simulink model "Simulink_Pendu_v1"  (R2019a)
settings: Solver=FixedStepAuto  StartTime=0.0  StopTime=inf  RelTol=1e-3  EnableMultiTasking=on
libraries: eeGeneralControl x3, cm_custom x2, simulink x1
settings Model: SimulationMode=external  Creator=Ng Wee Shen  LastModifiedBy=rng
settings SolverCC: PositivePriorityOrder=on  AutoInsertRateTranBlk=on
settings DataIOCC: ReturnWorkspaceOutputs=off
settings OptimizationCC: EnhancedBackFolding=on  PassReuseOutputArgsAs=Individual arguments  MaxStackSize=64  OptimizeBlockOrder=speed  DifferentSizesBufferReuse=on
settings DebuggingCC: TimeAdjustmentMsg=warning  SingleTaskRateTransMsg=warning  ParameterTunabilityLossMsg=error  SFcnCompatibilityMsg=warning  ArithmeticOperatorsInVariantConditions=warning
settings HardwareCC: ProdBitPerPointer=32  ProdBitPerSizeT=32  ProdBitPerPtrDiffT=32  ProdLargestAtomicInteger=Long  ProdLargestAtomicFloat=Double  ProdWordSize=32  ProdHWDeviceType=ARM Compatible->ARM Cortex
settings SFSimCC: MATLABDynamicMemAlloc=off
settings RTWCC: SystemTargetFile=ert.tlc  HardwareBoard=Raspberry Pi  TLCOptions="-aInlineSetEventsForThisBaseRateFcn=TLC_FALSE -aSuppressMultiTaskScheduler=TLC_FALSE  -aRateBasedStepFcn=0"  TemplateMakefile=ert_default_tmf  Toolchain=GNU GCC Raspberry Pi  BuildConfiguration=Specify  IncludeHyperlinkInReport=on  TargetLang=C++
settings CodeAppCC: ForceParamTrailComments=on  IgnoreCustomStorageClasses=off  OperatorAnnotations=on  SimulinkDataObjDesc=on  SFDataObjDesc=on  InsertBlockDesc=on
settings ERTTargetCC: TargetLangStandard=C++03 (ISO)  SupportContinuousTime=on  SupportVariableSizeSignals=on  ExtMode=on  ExtModeMexArgs='192.168.0.173' 1 17725

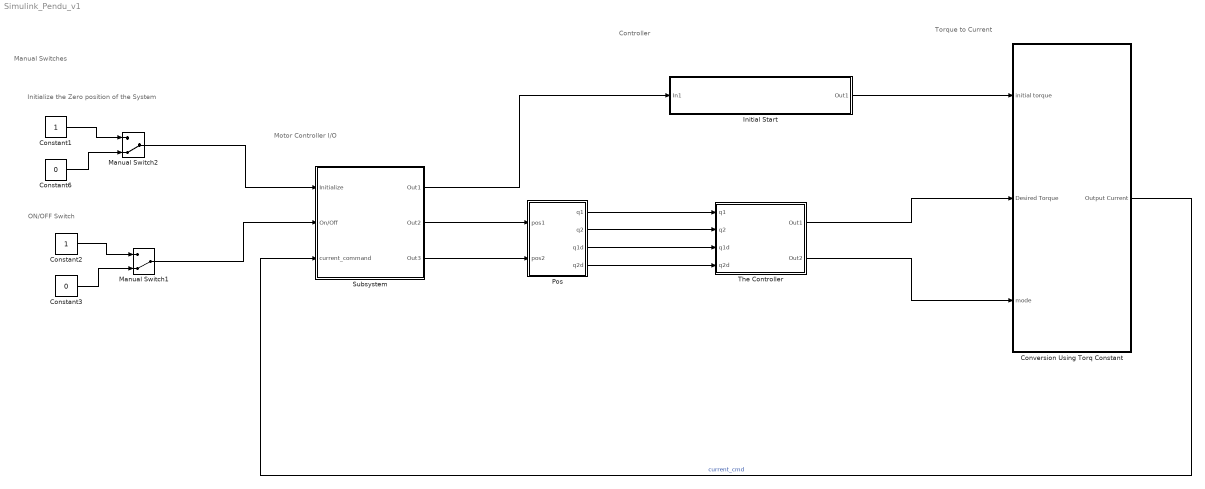
== system Simulink_Pendu_v1 ==
  note: Torque to Current
  note: Controller
  note: Motor Controller I/O
  note: Manual Switches
  note: ON/OFF Switch
  note: Initialize the Zero position of the System
  Constant1 : Constant
  Constant2 : Constant
  Constant3 : Constant  Value=0
  Constant6 : Constant  Value=0
  Conversion Using Torq Constant : Subsystem
  Initial Start : Subsystem
  Manual Switch1 : ManualSwitch  CurrentSetting=0
  Manual Switch2 : ManualSwitch  CurrentSetting=0
  Pos : Subsystem
  Subsystem : Subsystem
  The Controller : Subsystem
  wires:
  Constant1/1 -> Manual Switch2/1
  Constant6/1 -> Manual Switch2/2
  Initial Start/1(Out1) -> Conversion Using Torq Constant/1(initial torque)
  Pos/1(q1) -> The Controller/1(q1)
  Pos/2(q2) -> The Controller/2(q2)
  Pos/3(q1d) -> The Controller/3(q1d)
  Pos/4(q2d) -> The Controller/4(q2d)
  The Controller/1(Out1) -> Conversion Using Torq Constant/2(Desired Torque)
  The Controller/2(Out2) -> Conversion Using Torq Constant/3(" mode ")
  Manual Switch2/1 -> Subsystem/1(Initialize)
  Subsystem/1(Out1) -> Initial Start/1(In1)
  Subsystem/2(Out2) -> Pos/1(pos1)
  Subsystem/3(Out3) -> Pos/2(pos2)
  Constant2/1 -> Manual Switch1/1
  Constant3/1 -> Manual Switch1/2
  Manual Switch1/1 -> Subsystem/2(On/Off)
  Conversion Using Torq Constant/1(Output Current) -> Subsystem/3(current_command)  "current_cmd"

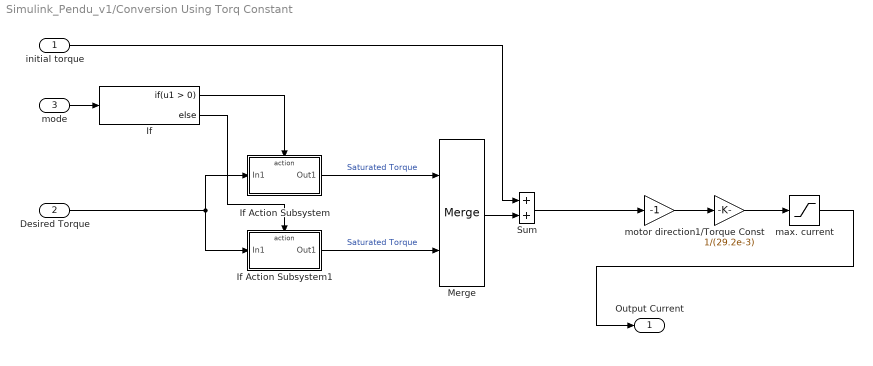
== system Simulink_Pendu_v1/Conversion Using Torq Constant ==
  initial torque : Inport
  Desired Torque : Inport  Port=2
  " mode " : Inport  Port=3
  1/Torque Const : Gain  Gain=1/(29.2e-3)  OutDataTypeStr=Inherit: Same as input
  If : If
  If Action Subsystem : Subsystem  TreatAsAtomicUnit=on
  If Action Subsystem1 : Subsystem  TreatAsAtomicUnit=on
  Merge : Merge
  Sum : Sum
  max. current : Saturate  UpperLimit=3  LowerLimit=-3  LinearizeAsGain=off
  motor direction : Gain  Gain=-1  OutDataTypeStr=Inherit: Same as input
  Output Current : Outport
  wires:
  motor direction/1 -> 1/Torque Const/1
  1/Torque Const/1 -> max. current/1
  " mode "/1 -> If/1
  Desired Torque/1 -> If Action Subsystem/1(In1), If Action Subsystem1/1(In1)
  If Action Subsystem/1(Out1) -> Merge/1  "Saturated Torque"
  If Action Subsystem1/1(Out1) -> Merge/2  "Saturated Torque"
  If/1 -> If Action Subsystem/Action
  If/2 -> If Action Subsystem1/Action
  Merge/1 -> Sum/2
  Sum/1 -> motor direction/1
  initial torque/1 -> Sum/1
  max. current/1 -> Output Current/1

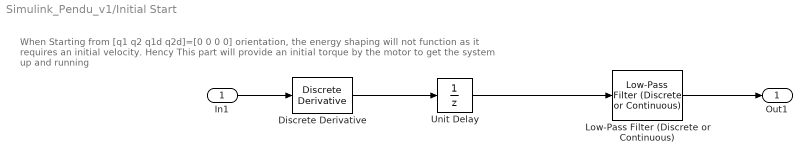
== system Simulink_Pendu_v1/Initial Start ==
  note: When Starting from [q1 q2 q1d q2d]=[0 0 0 0] orientation, the energy shaping will not function as it requires an initial velocity. Hency This part will provide an initial torque by the motor to get the system up and running
  In1 : Inport
  Discrete Derivative : simulink/Discrete/Discrete Derivative  gainval=1.0  ICPrevScaledInput=0.0  OutMin=[]  OutMax=[]  OutDataType=fixdt(1, 16)  OutScaling=2^-10  DoSatur=off
  Low-Pass Filter (Discrete or Continuous) : eeGeneralControl/Low-Pass Filter (Discrete or Continuous)  K=-1  T=0.025  B=0.05  A=-0.05  Ts=-1
      settings: SourceProductName=Simscape Electrical
  Unit Delay : UnitDelay  SampleTime=-1  HasFrameUpgradeWarning=on
  Out1 : Outport
  wires:
  Discrete Derivative/1 -> Unit Delay/1
  Unit Delay/1 -> Low-Pass Filter (Discrete or Continuous)/1
  Low-Pass Filter (Discrete or Continuous)/1 -> Out1/1
  In1/1 -> Discrete Derivative/1

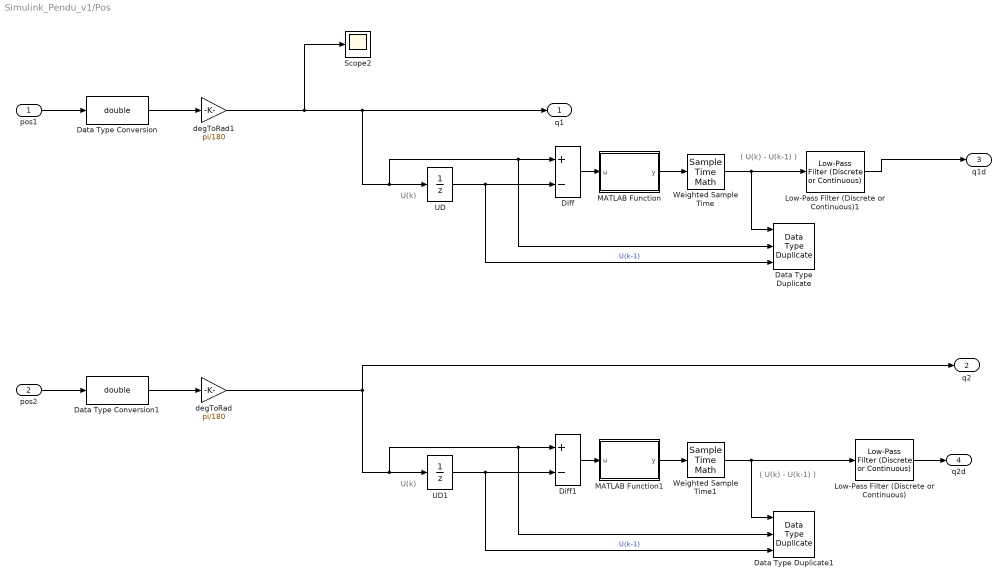
== system Simulink_Pendu_v1/Pos ==
  note: ( U(k) - U(k-1) )
  note: U(k)
  note: U(k)
  note: ( U(k) - U(k-1) )
  pos1 : Inport
  pos2 : Inport  Port=2
  Data Type Duplicate : DataTypeDuplicate  DisableCoverage=on  NumInputPorts=3
  Data Type Duplicate1 : DataTypeDuplicate  DisableCoverage=on  NumInputPorts=3
  Data Type Conversion : DataTypeConversion  OutDataTypeStr=double
  Data Type Conversion1 : DataTypeConversion  OutDataTypeStr=double
  Diff : Sum  Description=Add in CPU  Inputs=+-
  Diff1 : Sum  Description=Add in CPU  Inputs=+-
  Low-Pass Filter (Discrete or Continuous) : eeGeneralControl/Low-Pass Filter (Discrete or Continuous)  K=1  T=0.01  B=inf  A=-inf  Ts=-1
      settings: SourceProductName=Simscape Electrical
  Low-Pass Filter (Discrete or Continuous)1 : eeGeneralControl/Low-Pass Filter (Discrete or Continuous)  K=1  T=0.01  B=inf  A=-inf  Ts=-1
      settings: SourceProductName=Simscape Electrical
  MATLAB Function : MATLAB Function  TreatAsAtomicUnit=on
  MATLAB Function1 : MATLAB Function  TreatAsAtomicUnit=on
  Scope2 : Scope
  UD : UnitDelay  Description=Store in Global RAM  DisableCoverage=on  SampleTime=-1  HasFrameUpgradeWarning=on
  UD1 : UnitDelay  Description=Store in Global RAM  DisableCoverage=on  SampleTime=-1  HasFrameUpgradeWarning=on
  Weighted Sample Time : SampleTimeMath  TsampMathOp=/
  Weighted Sample Time1 : SampleTimeMath  TsampMathOp=/
  degToRad : Gain  Gain=pi/180
  degToRad1 : Gain  Gain=pi/180
  q1 : Outport
  q2 : Outport  Port=2
  q1d : Outport  Port=3
  q2d : Outport  Port=4
  wires:
  pos2/1 -> Data Type Conversion1/1
  pos1/1 -> Data Type Conversion/1
  Data Type Conversion1/1 -> degToRad/1
  Data Type Conversion/1 -> degToRad1/1
  Diff/1 -> MATLAB Function/1(u)
  UD/1 -> Diff/2, Data Type Duplicate/3  "U(k-1)"
  MATLAB Function/1(y) -> Weighted Sample Time/1
  Weighted Sample Time/1 -> Data Type Duplicate/1, Low-Pass Filter (Discrete or Continuous)1/1
  UD1/1 -> Diff1/2, Data Type Duplicate1/3  "U(k-1)"
  Diff1/1 -> MATLAB Function1/1(u)
  MATLAB Function1/1(y) -> Weighted Sample Time1/1
  Weighted Sample Time1/1 -> Data Type Duplicate1/1, Low-Pass Filter (Discrete or Continuous)/1
  degToRad1/1 -> Scope2/1, q1/1, UD/1, Diff/1, Data Type Duplicate/2
  Low-Pass Filter (Discrete or Continuous)/1 -> q2d/1
  Low-Pass Filter (Discrete or Continuous)1/1 -> q1d/1
  degToRad/1 -> q2/1, UD1/1, Diff1/1, Data Type Duplicate1/2

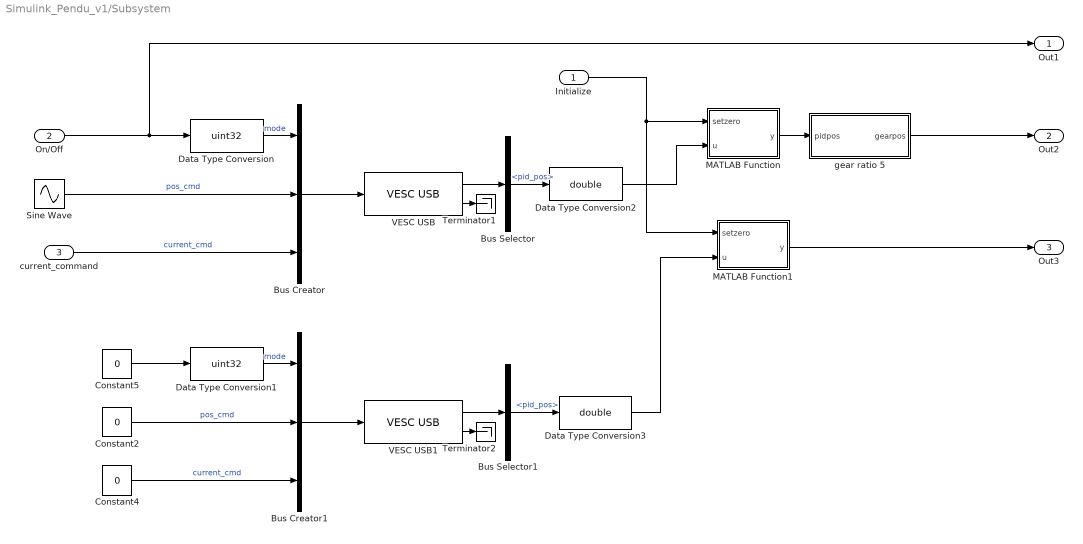
== system Simulink_Pendu_v1/Subsystem ==
  Initialize : Inport
  On/Off : Inport  Port=2
  current_command : Inport  Port=3
  Bus Creator : BusCreator  Inputs=3
  Bus Creator1 : BusCreator  Inputs=3
  Bus Selector : BusSelector  OutputSignals=pid_pos
  Bus Selector1 : BusSelector  OutputSignals=pid_pos
  Constant2 : Constant  Value=0
  Constant4 : Constant  Value=0
  Constant5 : Constant  Value=0
  Data Type Conversion : DataTypeConversion  OutDataTypeStr=uint32
  Data Type Conversion1 : DataTypeConversion  OutDataTypeStr=uint32
  Data Type Conversion2 : DataTypeConversion  OutDataTypeStr=double
  Data Type Conversion3 : DataTypeConversion  OutDataTypeStr=double
  MATLAB Function : MATLAB Function  TreatAsAtomicUnit=on
  MATLAB Function1 : MATLAB Function  TreatAsAtomicUnit=on
  Sine Wave : Sin  Amplitude=150  Bias=10  SampleTime=0
  Terminator1 : Terminator
  Terminator2 : Terminator
  VESC USB : cm_custom/VESC USB  PAR_VESC_DEV='/dev/USB_VESC2'  POS_KP=0.03  POS_KI=0  POS_KD=0.0004  POS_KD_FIL=0.2  POS_DIV=1  CURR_MAX=6  CURR_MIN=-6  CURR_IN_MAX=99  CURR_IN_MIN=-60  CURR_ABS_MAX=130  PAR_SMPLT=0.001
      settings: SourceProductName=cm custom
  VESC USB1 : cm_custom/VESC USB  PAR_VESC_DEV='/dev/USB_VESC1'  POS_KP=0.001  POS_KI=0  POS_KD=0.001  POS_KD_FIL=0.2  POS_DIV=1  CURR_MAX=20  CURR_MIN=-20  CURR_IN_MAX=20  CURR_IN_MIN=-20  CURR_ABS_MAX=20  PAR_SMPLT=0.001
      settings: SourceProductName=cm custom
  gear ratio 5 : Subsystem
  Out1 : Outport
  Out2 : Outport  Port=2
  Out3 : Outport  Port=3
  wires:
  Bus Selector1/1 -> Data Type Conversion3/1  "<pid_pos>"
  Bus Creator1/1 -> VESC USB1/1
  Data Type Conversion3/1 -> MATLAB Function1/2(u)
  Data Type Conversion1/1 -> Bus Creator1/1  "mode"
  VESC USB/1 -> Bus Selector/1
  Sine Wave/1 -> Bus Creator/2  "pos_cmd"
  Bus Selector/1 -> Data Type Conversion2/1  "<pid_pos>"
  VESC USB1/2 -> Terminator2/1
  VESC USB/2 -> Terminator1/1
  Bus Creator/1 -> VESC USB/1
  Data Type Conversion2/1 -> MATLAB Function/2(u)
  Constant2/1 -> Bus Creator1/2  "pos_cmd"
  Constant5/1 -> Data Type Conversion1/1
  Initialize/1 -> MATLAB Function1/1(setzero), MATLAB Function/1(setzero)
  VESC USB1/1 -> Bus Selector1/1
  Constant4/1 -> Bus Creator1/3  "current_cmd"
  MATLAB Function/1(y) -> gear ratio 5/1(pidpos)
  Data Type Conversion/1 -> Bus Creator/1  "mode"
  gear ratio 5/1(gearpos) -> Out2/1
  MATLAB Function1/1(y) -> Out3/1
  On/Off/1 -> Out1/1, Data Type Conversion/1
  current_command/1 -> Bus Creator/3  "current_cmd"

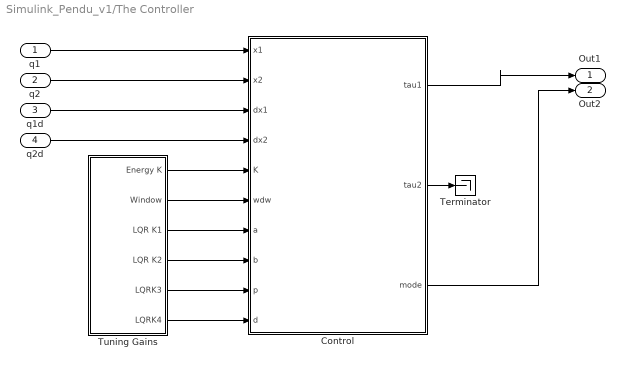
== system Simulink_Pendu_v1/The Controller ==
  q1 : Inport
  q2 : Inport  Port=2
  q1d : Inport  Port=3
  q2d : Inport  Port=4
  Control : MATLAB Function  TreatAsAtomicUnit=on
  Terminator : Terminator
  Tuning Gains : Subsystem
  Out1 : Outport
  Out2 : Outport  Port=2
  wires:
  q2d/1 -> Control/4(dx2)
  q1/1 -> Control/1(x1)
  Control/3(mode) -> Out2/1
  Tuning Gains/3(LQR K1) -> Control/7(a)
  Tuning Gains/5(LQRK3) -> Control/9(p)
  Tuning Gains/4(LQR K2) -> Control/8(b)
  Tuning Gains/6(LQRK4) -> Control/10(d)
  Tuning Gains/2(Window) -> Control/6(wdw)
  Control/2(tau2) -> Terminator/1
  Tuning Gains/1(Energy K) -> Control/5(K)
  Control/1(tau1) -> Out1/1
  q1d/1 -> Control/3(dx1)
  q2/1 -> Control/2(x2)

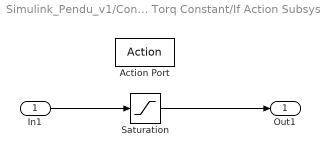
== system Simulink_Pendu_v1/Conversion Using Torq Constant/If Action Subsystem ==
  In1 : Inport
  Action Port : ActionPort  ActionPortLabel=if { }
  Saturation : Saturate  UpperLimit=0.055  LowerLimit=-0.055
  Out1 : Outport
  wires:
  In1/1 -> Saturation/1
  Saturation/1 -> Out1/1

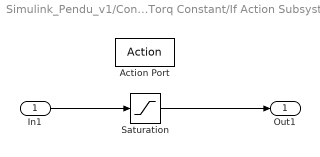
== system Simulink_Pendu_v1/Conversion Using Torq Constant/If Action Subsystem1 ==
  In1 : Inport
  Action Port : ActionPort  ActionPortLabel=else { }
  Saturation : Saturate  UpperLimit=0.035  LowerLimit=-0.035
  Out1 : Outport
  wires:
  In1/1 -> Saturation/1
  Saturation/1 -> Out1/1

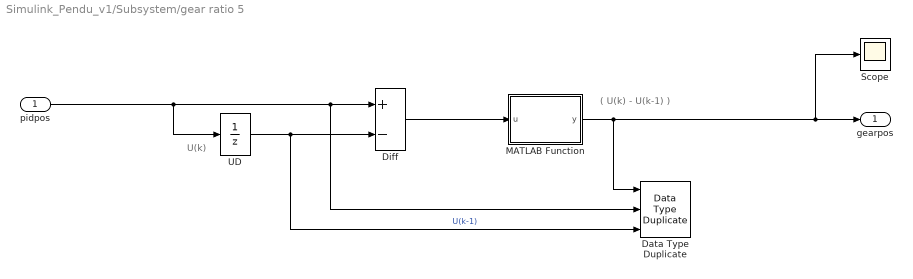
== system Simulink_Pendu_v1/Subsystem/gear ratio 5 ==
  note: ( U(k) - U(k-1) )
  note: U(k)
  pidpos : Inport
  Data Type Duplicate : DataTypeDuplicate  DisableCoverage=on  NumInputPorts=3
  Diff : Sum  Description=Add in CPU  Inputs=+-
  MATLAB Function : MATLAB Function  TreatAsAtomicUnit=on
  Scope : Scope
  UD : UnitDelay  Description=Store in Global RAM  DisableCoverage=on  SampleTime=-1  HasFrameUpgradeWarning=on
  gearpos : Outport
  wires:
  UD/1 -> Diff/2, Data Type Duplicate/3  "U(k-1)"
  pidpos/1 -> UD/1, Diff/1, Data Type Duplicate/2
  MATLAB Function/1(y) -> Data Type Duplicate/1, Scope/1, gearpos/1
  Diff/1 -> MATLAB Function/1(u)

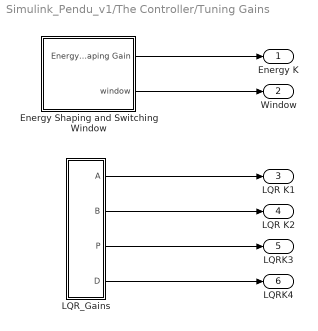
== system Simulink_Pendu_v1/The Controller/Tuning Gains ==
  Energy Shaping and Switching Window : Subsystem
  LQR_Gains : Subsystem
  Energy K : Outport
  Window : Outport  Port=2
  LQR K1 : Outport  Port=3
  LQR K2 : Outport  Port=4
  LQRK3 : Outport  Port=5
  LQRK4 : Outport  Port=6
  wires:
  LQR_Gains/3(P) -> LQRK3/1
  Energy Shaping and Switching Window/2(window) -> Window/1
  LQR_Gains/4(D) -> LQRK4/1
  Energy Shaping and Switching Window/1(EnergyShaping Gain) -> Energy K/1
  LQR_Gains/2(B) -> LQR K2/1
  LQR_Gains/1(A) -> LQR K1/1

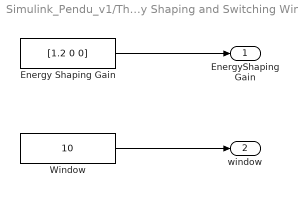
== system Simulink_Pendu_v1/The Controller/Tuning Gains/Energy Shaping and Switching Window ==
  Energy Shaping Gain : Constant  Value=[1.2 0 0]
  Window : Constant  Value=10
  EnergyShaping Gain : Outport
  window : Outport  Port=2
  wires:
  Energy Shaping Gain/1 -> EnergyShaping Gain/1
  Window/1 -> window/1

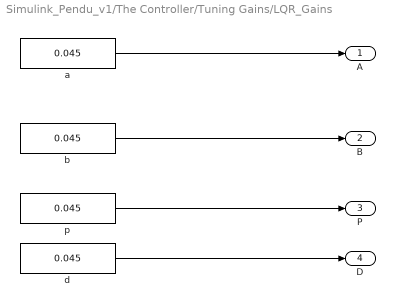
== system Simulink_Pendu_v1/The Controller/Tuning Gains/LQR_Gains ==
  a : Constant  Value=0.045
  b : Constant  Value=0.045
  d : Constant  Value=0.045
  p : Constant  Value=0.045
  A : Outport
  B : Outport  Port=2
  P : Outport  Port=3
  D : Outport  Port=4
  wires:
  p/1 -> P/1
  b/1 -> B/1
  d/1 -> D/1
  a/1 -> A/1

== matlab function Simulink_Pendu_v1/Subsystem/MATLAB Function ==
  data: setzero input; u input; y output
function y = fcn(setzero,u)

persistent initpos
if isempty(initpos)
    initpos = 0;
end

if setzero
    initpos = u + 0;
end


y = u - initpos;
y = y - 360*floor(y/360);

== matlab function Simulink_Pendu_v1/The Controller/Control ==
  data: x1 input; tau1 output; x2 input; dx1 input; dx2 input; K input; wdw input; a input; b input; p input; d input; tau2 output; mode output
function [tau1,tau2,mode] = EnergyShaping_w_LQR(x1,x2,dx1,dx2,K,wdw,a,b,p,d)
% Match the setup in simulation
x = [x1;x2;dx1;dx2]; 

persistent model;
if isempty(model)
    model = Model();
end

%%%%
q  = x(1:2,:);
qd = x(3:4,:);

[tau,mode] = acrobotControlLaw_LQR(x,wdw,a,b,p,d);

if isempty(tau) % if LQR control law is not applicable, 
                %    then using Energy Shaping approach
    mode = 0;
    g  = model.g;
    %
    l1 = model.l1; lc1 = model.lc1; l2 = model.l2; lc2 = model.lc2;
    m1 = model.m1; m2 = model.m2;
    I1 = model.I1; I2 = model.I2;
    b1 = model.b1; b2 = model.b2;

    %%%%
    q  = x(1:2,:);
    qd = x(3:4,:);

    %%%%
    c = cos(q(1:2,:));  s = sin(q(1:2,:));  c12 = cos(q(1,:)+q(2,:));
    
    [M,~] = ManipulatorEquation(model, x);
    %%%% energy shaping
    E_des = m1.*g.* lc1 + m2.*g.*(l1+lc2);

    KE = 0.5*qd.'*M*qd;
    PE = -m1*g*lc1*c(1) - m2*g*(l1*c(1)+lc2*c12);
    E = KE + PE;

    E_tilda = E_des - E;

%     ke = 1;    %0.75  %5   %0.05;
%     kd = 0*ke/10;  %25   %ke/15;
%     ks = 0*kd/5;   %8   %kd/10;
    ke = K(1);
    kd = K(2)*ke;
    ks = K(3)*kd;
    
    q(1) = q(1) - 2*pi*floor(q(1)./(2*pi));
    d_tilda = pi-q(1);
    s_tilda = 0-qd(1);
    
    % P-saturation
    PD = d_tilda*kd + s_tilda*ks;
    if abs(PD) > 1
        PD = 1 * sign(PD);
    end
    
    tau = [(ke.*E_tilda.*qd(1)+PD); 0]; 
    %tau = [(0); 0]; 
    
end
tau=(18/90)*tau;
tau1 = tau(1);

tau2 = tau(2);
end

== matlab function Simulink_Pendu_v1/Subsystem/MATLAB Function1 ==
  data: setzero input; u input; y output
function y = fcn(setzero,u)

persistent initpos
if isempty(initpos)
    initpos = 0;
end

if setzero
    initpos = u + 0;
end


y = u - initpos;
y = y - 360*floor(y/360);

== matlab function Simulink_Pendu_v1/Pos/MATLAB Function ==
  data: u input; y output
function y = fcn(u)

u_rev = (u >= 0)*(2*pi - u) + (u < 0)*(2*pi + u);

if abs(u_rev) > abs(u)
   y = u;
else
   y = (u < 0)*u_rev - (u >= 0)*u_rev;
end

== matlab function Simulink_Pendu_v1/Pos/MATLAB Function1 ==
  data: u input; y output
function y = fcn(u)

u_rev = (u >= 0)*(2*pi - u) + (u < 0)*(2*pi + u);

if abs(u_rev) > abs(u)
   y = u;
else
   y = (u < 0)*u_rev - (u >= 0)*u_rev;
end

== matlab function Simulink_Pendu_v1/Subsystem/gear ratio 5/MATLAB Function ==
  data: u input; y output
function y = fcn(u)

persistent pos1
if isempty(pos1)
    pos1 = 0;
end

u_rev = (u >= 0)*(360 - u) + (u < 0)*(360 + u);
if abs(u_rev) < abs(u)
   u = (u < 0)*u_rev - (u >= 0)*u_rev;
end

u = u/5;
pos1 = pos1 + u;
pos1 = mod((pos1),360);
y = pos1;

end
